simulink library "HV_CAN"  (R2017a)
settings: Solver=VariableStepAuto  StartTime=0.0  StopTime=10.0  RelTol=1e-3
settings Model: Creator=Di Russo  LastModifiedBy=Vraj M

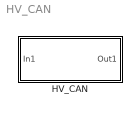
== system HV_CAN ==
  HV_CAN : Subsystem

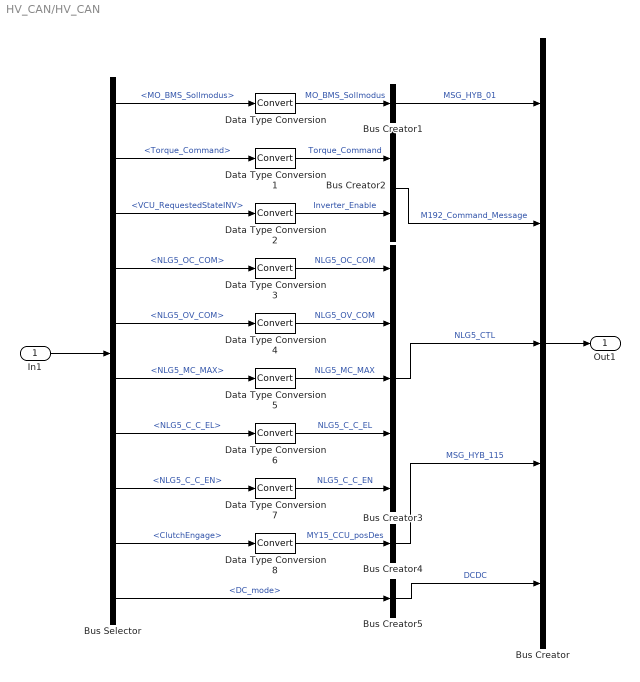
== system HV_CAN/HV_CAN ==
  In1 : Inport
  Bus Creator : BusCreator  Inputs=5
  Bus Creator1 : BusCreator  Inputs=1
  Bus Creator2 : BusCreator  Inputs=2
  Bus Creator3 : BusCreator  Inputs=5
  Bus Creator4 : BusCreator  Inputs=1
  Bus Creator5 : BusCreator  Inputs=1
  Bus Selector : BusSelector  OutputSignals=BMS_CAN.MSG_HYB_01.MO_BMS_Sollmodus,Controls.Torque_Command,MCU_CAN.MCU_CAN.VCU_RequestedStateINV,OBC_CAN.NLG5_OC_COM,OBC_CAN.NLG5_OV_COM,OBC_CAN.NLG5_MC_MAX,OBC_CAN.NLG5_C_C_EL,OBC_CAN.NLG5_C_C_EN,Controls.ClutchEngage,MCU_CAN.DCDC_Out.DC_mode
  Data Type Conversion{,1..8} (9 alike) : DataTypeConversion
  Out1 : Outport
  wires:
  Bus Creator5/1 -> Bus Creator/5  "DCDC"
  Bus Selector/10 -> Bus Creator5/1  "<DC_mode>"
  Bus Creator4/1 -> Bus Creator/4  "MSG_HYB_115"
  Data Type Conversion8/1 -> Bus Creator4/1  "MY15_CCU_posDes"
  Data Type Conversion7/1 -> Bus Creator3/5  "NLG5_C_C_EN"
  Data Type Conversion6/1 -> Bus Creator3/4  "NLG5_C_C_EL"
  Data Type Conversion5/1 -> Bus Creator3/3  "NLG5_MC_MAX"
  Data Type Conversion4/1 -> Bus Creator3/2  "NLG5_OV_COM"
  Data Type Conversion3/1 -> Bus Creator3/1  "NLG5_OC_COM"
  Bus Creator3/1 -> Bus Creator/3  "NLG5_CTL"
  Data Type Conversion2/1 -> Bus Creator2/2  "Inverter_Enable"
  Data Type Conversion1/1 -> Bus Creator2/1  "Torque_Command"
  Bus Selector/9 -> Data Type Conversion8/1  "<ClutchEngage>"
  Bus Selector/8 -> Data Type Conversion7/1  "<NLG5_C_C_EN>"
  Bus Selector/7 -> Data Type Conversion6/1  "<NLG5_C_C_EL>"
  Bus Selector/6 -> Data Type Conversion5/1  "<NLG5_MC_MAX>"
  Bus Selector/5 -> Data Type Conversion4/1  "<NLG5_OV_COM>"
  Bus Selector/4 -> Data Type Conversion3/1  "<NLG5_OC_COM>"
  Bus Creator2/1 -> Bus Creator/2  "M192_Command_Message"
  Bus Selector/3 -> Data Type Conversion2/1  "<VCU_RequestedStateINV>"
  Bus Selector/2 -> Data Type Conversion1/1  "<Torque_Command>"
  Bus Creator1/1 -> Bus Creator/1  "MSG_HYB_01"
  Data Type Conversion/1 -> Bus Creator1/1  "MO_BMS_Sollmodus"
  Bus Selector/1 -> Data Type Conversion/1  "<MO_BMS_Sollmodus>"
  In1/1 -> Bus Selector/1
  Bus Creator/1 -> Out1/1
